simulink model "PassengerVehicle"  (R2018b)
settings: configuration reference "Physics" (kept outside this file)
model workspace (MAT data in the model file):
  m = 1000
undefined symbols (not defined in the file): brake_param, DiscIntNeverNeededParam, tSPhysics, TUMHealthStatus, veh_param, x0_positionstates, x0_vehiclepose
libraries: general_sensor_lib x20, misc x2
settings Model: DataDictionary=PassengerVehicle.sldd  PauseTimes=9.280  Creator=wischnewski  LastModifiedBy=ga25xiw

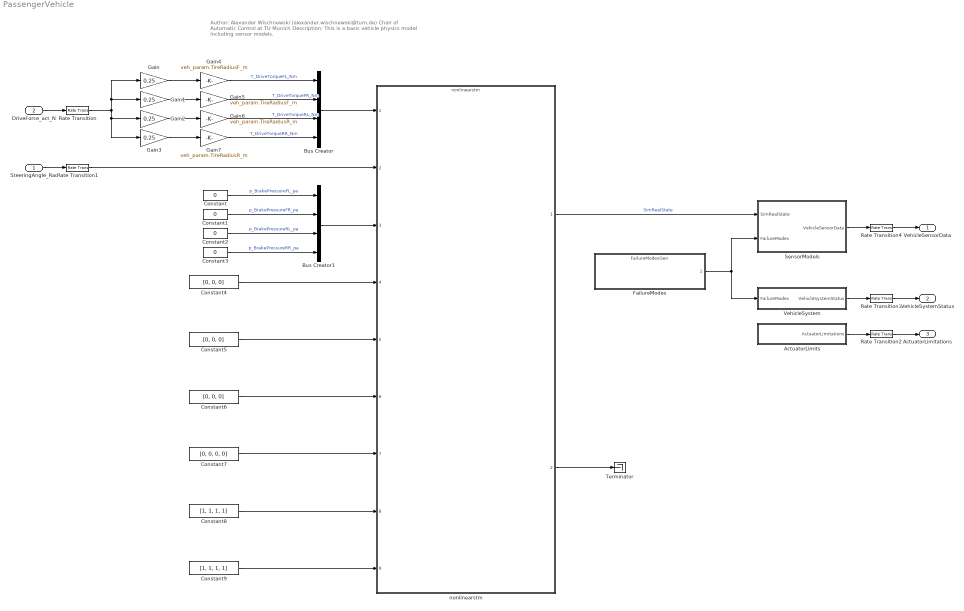
== system PassengerVehicle ==
  note: Author: Alexander Wischnewski (alexander.wischnewski@tum.de)
      | Chair of Automatic Control at TU Munich
      |
      | Description: This is a basic vehicle physics model including sensor models.
  SteeringAngle_Rad : Inport
  DriveForce_act_N : Inport  Port=2
  ActuatorLimits : Subsystem
  Bus Creator : BusCreator  Inputs=4
  Bus Creator1 : BusCreator  Inputs=4
  Constant{,1..3} (4 alike) : Constant  Value=0
  Constant4 : Constant  Value=[0, 0, 0]
  Constant5 : Constant  Value=[0, 0, 0]
  Constant6 : Constant  Value=[0, 0, 0]
  Constant7 : Constant  Value=[0, 0, 0, 0]
  Constant8 : Constant  Value=[1, 1, 1, 1]
  Constant9 : Constant  Value=[1, 1, 1, 1]
  FailureModes : ModelReference  ModelNameDialog=FailureModesGen  SimulationMode=Normal  ModelReferenceVersion=1.709
  Gain{,1..3} (4 alike) : Gain  Gain=0.25
  Gain4 : Gain  Gain=veh_param.TireRadiusF_m
  Gain5 : Gain  Gain=veh_param.TireRadiusF_m
  Gain6 : Gain  Gain=veh_param.TireRadiusR_m
  Gain7 : Gain  Gain=veh_param.TireRadiusR_m
  Rate Transition{,1..4} (5 alike) : RateTransition
  SensorModels : Subsystem
  Terminator : Terminator
  VehicleSystem : Subsystem
  nonlinearstm : ModelReference  ModelNameDialog=nonlinearstm.slx  ParameterArgumentNames=brake_param,veh_param,x0_positionstates  ParameterArgumentValues=brake_param,veh_param,x0_vehiclepose  UsingDefaultArgumentValue=0,0,0  SimulationMode=Normal  ModelReferenceVersion=1.335
  VehicleSensorData : Outport  OutDataTypeStr=Bus: VehicleSensorData
  VehicleSystemStatus : Outport  Port=2  OutDataTypeStr=Bus: VehicleSystemStatus
  ActuatorLimitations : Outport  Port=3  OutDataTypeStr=Bus: ActuatorLimitations
  wires:
  nonlinearstm/2 -> Terminator/1
  Gain2/1 -> Gain6/1
  Gain1/1 -> Gain5/1
  Constant8/1 -> nonlinearstm/8
  Constant9/1 -> nonlinearstm/9
  FailureModes/1 -> SensorModels/2(FailureModes), VehicleSystem/1(FailureModes)
  Rate Transition1/1 -> nonlinearstm/2
  Gain3/1 -> Gain7/1
  Constant2/1 -> Bus Creator1/3  "p_BrakePressureRL_pa"
  Constant3/1 -> Bus Creator1/4  "p_BrakePressureRR_pa"
  Constant7/1 -> nonlinearstm/7
  Constant/1 -> Bus Creator1/1  "p_BrakePressureFL_pa"
  Gain/1 -> Gain4/1
  Rate Transition4/1 -> VehicleSensorData/1
  Constant1/1 -> Bus Creator1/2  "p_BrakePressureFR_pa"
  Constant4/1 -> nonlinearstm/4
  Gain7/1 -> Bus Creator/4  "T_DriveTorqueRR_Nm"
  Constant6/1 -> nonlinearstm/6
  VehicleSystem/1(VehicleSystemStatus) -> Rate Transition3/1
  Gain6/1 -> Bus Creator/3  "T_DriveTorqueRL_Nm"
  Constant5/1 -> nonlinearstm/5
  nonlinearstm/1 -> SensorModels/1(SimRealState)  "SimRealState"
  Gain5/1 -> Bus Creator/2  "T_DriveTorqueFR_Nm"
  Gain4/1 -> Bus Creator/1  "T_DriveTorqueFL_Nm"
  Rate Transition/1 -> Gain1/1, Gain/1, Gain3/1, Gain2/1
  SensorModels/1(VehicleSensorData) -> Rate Transition4/1
  Bus Creator1/1 -> nonlinearstm/3
  Rate Transition3/1 -> VehicleSystemStatus/1
  Bus Creator/1 -> nonlinearstm/1
  Rate Transition2/1 -> ActuatorLimitations/1
  ActuatorLimits/1(ActuatorLimitations) -> Rate Transition2/1
  DriveForce_act_N/1 -> Rate Transition/1
  SteeringAngle_Rad/1 -> Rate Transition1/1

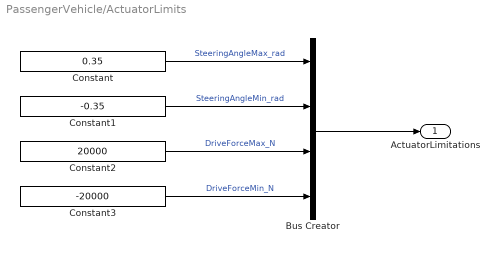
== system PassengerVehicle/ActuatorLimits ==
  Bus Creator : BusCreator  Inputs=4
  Constant : Constant  Value=0.35
  Constant1 : Constant  Value=-0.35
  Constant2 : Constant  Value=20000
  Constant3 : Constant  Value=-20000
  ActuatorLimitations : Outport
  wires:
  Bus Creator/1 -> ActuatorLimitations/1
  Constant/1 -> Bus Creator/1  "SteeringAngleMax_rad"
  Constant1/1 -> Bus Creator/2  "SteeringAngleMin_rad"
  Constant2/1 -> Bus Creator/3  "DriveForceMax_N"
  Constant3/1 -> Bus Creator/4  "DriveForceMin_N"

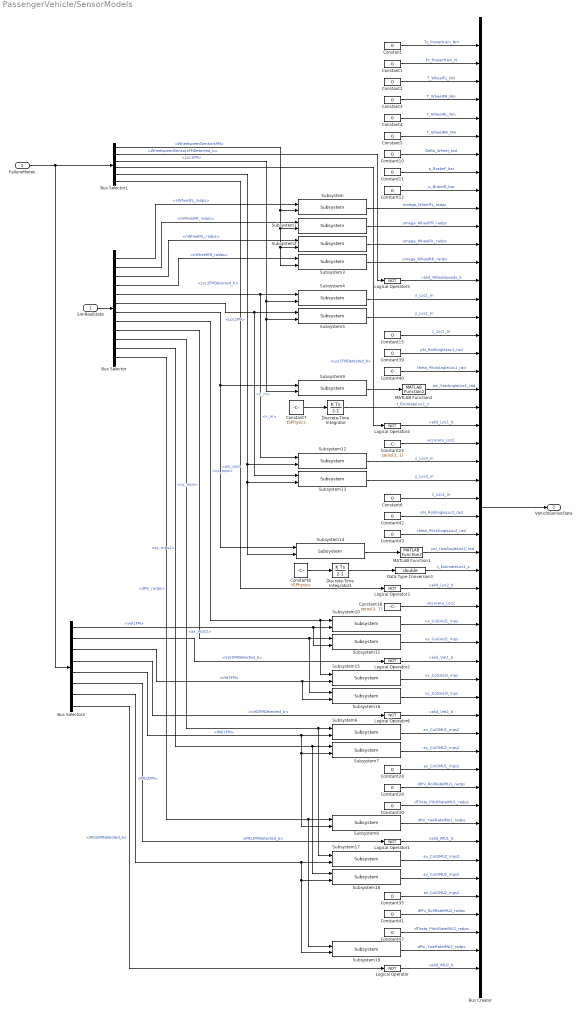
== system PassengerVehicle/SensorModels ==
  SimRealState : Inport
  FailureModes : Inport  Port=2
  Bus Creator : BusCreator  Inputs=52  OutDataTypeStr=Bus: VehicleSensorData
  Bus Selector : BusSelector  OutputSignals=nWheelFL_radps,nWheelFR_radps,nWheelRL_radps,nWheelRR_radps,x_m,y_m,psi_rad,vx_mps,vy_mps,ax_mps2,ay_mps2,dPsi_radps
  Bus Selector1 : BusSelector  OutputSignals=WheelspeedSensorsFM,WheelspeedSensorsFMDetected_b,Loc1FM,Loc1FMDetected_b,Loc2FM,Loc2FMDetected_b
  Bus Selector2 : BusSelector  OutputSignals=Vel1FM,Vel1FMDetected_b,Vel2FM,Vel2FMDetected_b,IMU1FM,IMU1FMDetected_b,IMU2FM,IMU2FMDetected_b
  Constant{,1..6,10..12,15,28..30,35,39..43,47} (21 alike) : Constant  Value=0
  Constant23 : Constant  Value=zeros(3, 1)
  Constant38 : Constant  Value=zeros(3, 1)
  Constant7 : Constant  Value=tSPhysics
  Constant8 : Constant  Value=tSPhysics
  Data Type Conversion1 : DataTypeConversion  OutDataTypeStr=double
  Discrete-Time Integrator : DiscreteIntegrator  SampleTime=tSPhysics  ICPrevOutput=DiscIntNeverNeededParam  ICPrevScaledInput=DiscIntNeverNeededParam
  Discrete-Time Integrator1 : DiscreteIntegrator  SampleTime=tSPhysics  ICPrevOutput=DiscIntNeverNeededParam  ICPrevScaledInput=DiscIntNeverNeededParam
  Logical Operator{,1..6} (7 alike) : Logic  Operator=NOT  Inputs=1  AllPortsSameDT=off  OutDataTypeStr=boolean
  MATLAB Function1 : misc/MATLAB Function2  SystemSampleTime=-1
  MATLAB Function2 : misc/MATLAB Function2  SystemSampleTime=-1
  Subsystem : general_sensor_lib/Subsystem  Noise=0.1  Delay=0  SampleRate=tSPhysics  seed=436
  Subsystem1 : general_sensor_lib/Subsystem  Noise=0.1  Delay=0  SampleRate=tSPhysics  seed=438
  Subsystem10 : general_sensor_lib/Subsystem  Noise=0.01  Delay=0  SampleRate=tSPhysics  seed=4577
  Subsystem11 : general_sensor_lib/Subsystem  Noise=0.01  Delay=0  SampleRate=tSPhysics  seed=127
  Subsystem12 : general_sensor_lib/Subsystem  Noise=0.001  Delay=0  SampleRate=tSPhysics  seed=237
  Subsystem13 : general_sensor_lib/Subsystem  Noise=0.001  Delay=0  SampleRate=tSPhysics  seed=327
  Subsystem14 : general_sensor_lib/Subsystem  Noise=0.001  Delay=0  SampleRate=tSPhysics  seed=347
  Subsystem15 : general_sensor_lib/Subsystem  Noise=0.01  Delay=0  SampleRate=tSPhysics  seed=459
  Subsystem16 : general_sensor_lib/Subsystem  Noise=0.01  Delay=0  SampleRate=tSPhysics  seed=467
  Subsystem17 : general_sensor_lib/Subsystem  Noise=0.05  Delay=0  SampleRate=tSPhysics  seed=37
  Subsystem18 : general_sensor_lib/Subsystem  Noise=0.05  Delay=0  SampleRate=tSPhysics  seed=0
  Subsystem19 : general_sensor_lib/Subsystem  Noise=0.0002  Delay=0  SampleRate=tSPhysics  seed=0
  Subsystem2 : general_sensor_lib/Subsystem  Noise=0.1  Delay=0  SampleRate=tSPhysics  seed=137
  Subsystem3 : general_sensor_lib/Subsystem  Noise=0.1  Delay=0  SampleRate=tSPhysics  seed=345
  Subsystem4 : general_sensor_lib/Subsystem  Noise=0.001  Delay=0  SampleRate=tSPhysics  seed=596
  Subsystem5 : general_sensor_lib/Subsystem  Noise=0.001  Delay=0  SampleRate=tSPhysics  seed=973
  Subsystem6 : general_sensor_lib/Subsystem  Noise=0.05  Delay=0  SampleRate=tSPhysics  seed=456
  Subsystem7 : general_sensor_lib/Subsystem  Noise=0.05  Delay=0  SampleRate=tSPhysics  seed=78
  Subsystem8 : general_sensor_lib/Subsystem  Noise=0.0002  Delay=0  SampleRate=tSPhysics  seed=43
  Subsystem9 : general_sensor_lib/Subsystem  Noise=0.001  Delay=0  SampleRate=tSPhysics  seed=578
  VehicleSensorData : Outport
  wires:
  Bus Creator/1 -> VehicleSensorData/1
  Constant/1 -> Bus Creator/1  "Tz_Powertrain_Nm"
  Constant1/1 -> Bus Creator/2  "Fx_Powertrain_N"
  Constant2/1 -> Bus Creator/3  "T_WheelFL_Nm"
  Constant3/1 -> Bus Creator/4  "T_WheelFR_Nm"
  Constant4/1 -> Bus Creator/5  "T_WheelRL_Nm"
  Constant5/1 -> Bus Creator/6  "T_WheelRR_Nm"
  Subsystem/1 -> Bus Creator/10  "omega_WheelFL_radps"
  Subsystem1/1 -> Bus Creator/11  "omega_WheelFR_radps"
  Subsystem2/1 -> Bus Creator/12  "omega_WheelRL_radps"
  Subsystem3/1 -> Bus Creator/13  "omega_WheelRR_radps"
  Constant10/1 -> Bus Creator/7  "Delta_Wheel_rad"
  Constant11/1 -> Bus Creator/8  "p_BrakeF_bar"
  Constant12/1 -> Bus Creator/9  "p_BrakeR_bar"
  Subsystem4/1 -> Bus Creator/15  "x_Loc1_m"
  Subsystem5/1 -> Bus Creator/16  "y_Loc1_m"
  Constant15/1 -> Bus Creator/17  "z_Loc1_m"
  Discrete-Time Integrator/1 -> Bus Creator/21  "t_EstimateLoc1_s"
  Subsystem12/1 -> Bus Creator/24  "x_Loc2_m"
  Subsystem13/1 -> Bus Creator/25  "y_Loc2_m"
  Constant6/1 -> Bus Creator/26  "z_Loc2_m"
  Logical Operator3/1 -> Bus Creator/31  "valid_Loc2_b"
  Subsystem6/1 -> Bus Creator/39  "ax_CoGIMU1_mps2"
  Subsystem7/1 -> Bus Creator/40  "ay_CoGIMU1_mps2"
  Constant28/1 -> Bus Creator/41  "az_CoGIMU1_mps2"
  Constant29/1 -> Bus Creator/42  "dPhi_RollRateIMU1_radps"
  Constant30/1 -> Bus Creator/43  "dTheta_PitchRateIMU1_radps"
  Subsystem8/1 -> Bus Creator/44  "dPsi_YawRateIMU1_radps"
  Subsystem9/1 -> MATLAB Function2/1
  SimRealState/1 -> Bus Selector/1
  Bus Selector/1 -> Subsystem/1  "<nWheelFL_radps>"
  Bus Selector/2 -> Subsystem1/1  "<nWheelFR_radps>"
  Bus Selector/3 -> Subsystem2/1  "<nWheelRL_radps>"
  Bus Selector/4 -> Subsystem3/1  "<nWheelRR_radps>"
  Bus Selector/5 -> Subsystem12/1, Subsystem4/1  "<x_m>"
  Bus Selector/6 -> Subsystem13/1, Subsystem5/1  "<y_m>"
  Bus Selector/10 -> Subsystem17/1, Subsystem6/1  "<ax_mps2>"
  Bus Selector/11 -> Subsystem18/1, Subsystem7/1  "<ay_mps2>"
  Bus Selector/12 -> Subsystem19/1, Subsystem8/1  "<dPsi_radps>"
  Bus Selector/8 -> Subsystem15/1, Subsystem10/1  "<vx_mps>"
  Bus Selector/9 -> Subsystem16/1, Subsystem11/1  "<vy_mps>"
  Bus Selector1/3 -> Subsystem9/2, Subsystem5/2, Subsystem4/2  "<Loc1FM>"
  Data Type Conversion1/1 -> Bus Creator/30  "t_EstimateLoc2_s"
  Bus Selector/7 -> Subsystem14/1, Subsystem9/1  "<psi_rad>"
  Constant23/1 -> Bus Creator/23  "accuracy_Loc1"
  Constant38/1 -> Bus Creator/32  "accuracy_Loc2"
  Constant39/1 -> Bus Creator/18  "phi_RollAngleLoc1_rad"
  Constant40/1 -> Bus Creator/19  "theta_PitchAngleLoc1_rad"
  MATLAB Function2/1 -> Bus Creator/20  "psi_YawAngleLoc1_rad"
  Constant42/1 -> Bus Creator/27  "phi_RollAngleLoc2_rad"
  Constant43/1 -> Bus Creator/28  "theta_PitchAngleLoc2_rad"
  MATLAB Function1/1 -> Bus Creator/29  "psi_YawAngleLoc2_rad"
  Subsystem10/1 -> Bus Creator/33  "vx_CoGVel1_mps"
  Subsystem11/1 -> Bus Creator/34  "vy_CoGVel1_mps"
  Subsystem15/1 -> Bus Creator/36  "vx_CoGVel2_mps"
  Subsystem16/1 -> Bus Creator/37  "vy_CoGVel2_mps"
  Subsystem17/1 -> Bus Creator/46  "ax_CoGIMU2_mps2"
  Subsystem18/1 -> Bus Creator/47  "ay_CoGIMU2_mps2"
  Constant35/1 -> Bus Creator/48  "az_CoGIMU2_mps2"
  Constant41/1 -> Bus Creator/49  "dPhi_RollRateIMU2_radps"
  Constant47/1 -> Bus Creator/50  "dTheta_PitchRateIMU2_radps"
  Subsystem19/1 -> Bus Creator/51  "dPsi_YawRateIMU2_radps"
  Logical Operator6/1 -> Bus Creator/38  "valid_Vel2_b"
  Logical Operator/1 -> Bus Creator/52  "valid_IMU2_b"
  Logical Operator1/1 -> Bus Creator/45  "valid_IMU1_b"
  Logical Operator2/1 -> Bus Creator/35  "valid_Vel1_b"
  Logical Operator5/1 -> Bus Creator/14  "valid_Wheelspeeds_b"
  FailureModes/1 -> Bus Selector2/1, Bus Selector1/1
  Bus Selector1/1 -> Subsystem3/2, Subsystem2/2, Subsystem1/2, Subsystem/2  "<WheelspeedSensorsFM>"
  Bus Selector1/2 -> Logical Operator5/1  "<WheelspeedSensorsFMDetected_b>"
  Logical Operator4/1 -> Bus Creator/22  "valid_Loc1_b"
  Bus Selector1/4 -> Logical Operator4/1  "<Loc1FMDetected_b>"
  Bus Selector2/1 -> Subsystem11/2, Subsystem10/2  "<Vel1FM>"
  Bus Selector2/2 -> Logical Operator2/1  "<Vel1FMDetected_b>"
  Bus Selector2/5 -> Subsystem8/2, Subsystem7/2, Subsystem6/2  "<IMU1FM>"
  Bus Selector2/6 -> Logical Operator1/1  "<IMU1FMDetected_b>"
  Subsystem14/1 -> MATLAB Function1/1
  Discrete-Time Integrator1/1 -> Data Type Conversion1/1
  Bus Selector1/5 -> Subsystem14/2, Subsystem13/2, Subsystem12/2  "<Loc2FM>"
  Bus Selector1/6 -> Logical Operator3/1  "<Loc2FMDetected_b>"
  Bus Selector2/3 -> Subsystem15/2, Subsystem16/2  "<Vel2FM>"
  Bus Selector2/4 -> Logical Operator6/1  "<Vel2FMDetected_b>"
  Bus Selector2/7 -> Subsystem19/2, Subsystem18/2, Subsystem17/2  "<IMU2FM>"
  Bus Selector2/8 -> Logical Operator/1  "<IMU2FMDetected_b>"
  Constant7/1 -> Discrete-Time Integrator/1
  Constant8/1 -> Discrete-Time Integrator1/1

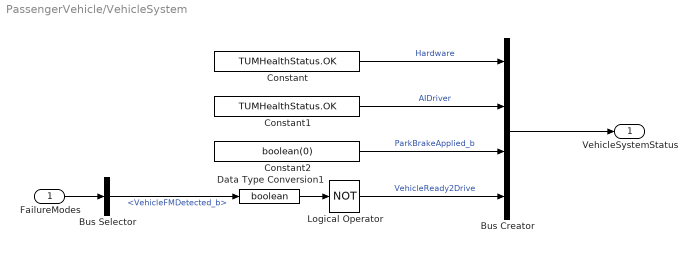
== system PassengerVehicle/VehicleSystem ==
  FailureModes : Inport
  Bus Creator : BusCreator  Inputs=4
  Bus Selector : BusSelector  OutputSignals=VehicleFMDetected_b
  Constant : Constant  Value=TUMHealthStatus.OK
  Constant1 : Constant  Value=TUMHealthStatus.OK
  Constant2 : Constant  Value=boolean(0)
  Data Type Conversion1 : DataTypeConversion  OutDataTypeStr=boolean
  Logical Operator : Logic  Operator=NOT  Inputs=1  AllPortsSameDT=off  OutDataTypeStr=boolean
  VehicleSystemStatus : Outport
  wires:
  Bus Creator/1 -> VehicleSystemStatus/1
  Constant/1 -> Bus Creator/1  "Hardware"
  Constant1/1 -> Bus Creator/2  "AIDriver"
  Constant2/1 -> Bus Creator/3  "ParkBrakeApplied_b"
  Logical Operator/1 -> Bus Creator/4  "VehicleReady2Drive"
  Data Type Conversion1/1 -> Logical Operator/1
  FailureModes/1 -> Bus Selector/1
  Bus Selector/1 -> Data Type Conversion1/1  "<VehicleFMDetected_b>"
